simulink model "SpoolWrap"  (R2013b)
settings: Solver=ode3  StartTime=0.0  StopTime=5  FixedStep=.001  RelTol=1e-3
libraries: simulink x3
settings Model: Creator=LukePH  LastModifiedBy=LukePH

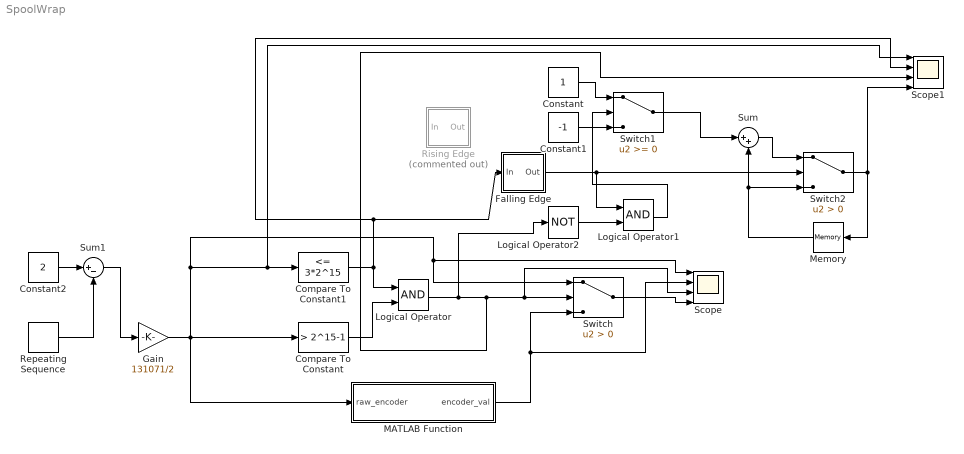
== system SpoolWrap ==
  Compare To Constant : simulink/Logic and Bit Operations/Compare To Constant  relop=>  const=2^15-1  OutDataTypeStr=boolean
  Compare To Constant1 : simulink/Logic and Bit Operations/Compare To Constant  relop=<=  const=3*2^15  OutDataTypeStr=boolean
  Constant : Constant
  Constant1 : Constant  Value=-1
  Constant2 : Constant  Value=2
  Falling Edge : Subsystem
  Gain : Gain  Gain=131071/2  OutDataTypeStr=int32
  Logical Operator : Logic  AllPortsSameDT=off  OutDataTypeStr=boolean
  Logical Operator1 : Logic  AllPortsSameDT=off  OutDataTypeStr=boolean
  Logical Operator2 : Logic  Operator=NOT  AllPortsSameDT=off  OutDataTypeStr=boolean
  MATLAB Function : MATLAB Function  TreatAsAtomicUnit=on
  Memory : Memory
  Repeating Sequence : simulink/Sources/Repeating Sequence  rep_seq_t=[0 1]  rep_seq_y=[0 2]
  Rising Edge : Subsystem  Commented=on
  Scope : Scope  NumInputPorts=4
      settings: TimeRange=4  YMin=0~-70000~0~-40000  YMax=140000~70000~1~100000
  Scope1 : Scope  NumInputPorts=4
      settings: TimeRange=4  YMin=0~-5~-5~-5  YMax=140000~5~5~5
  Sum : Sum  Inputs=|++
  Sum1 : Sum  Inputs=|+-
  Switch : Switch  Criteria=u2 > Threshold
  Switch1 : Switch
  Switch2 : Switch  Criteria=u2 > Threshold
  wires:
  Repeating Sequence/1 -> Sum1/2
  Gain/1 -> Scope/1, Switch/1, Scope1/1, Compare To Constant1/1, Compare To Constant/1, MATLAB Function/1(raw_encoder)
  Compare To Constant/1 -> Logical Operator/2
  Switch/1 -> Scope/4
  MATLAB Function/1(encoder_val) -> Scope/2, Switch/3
  Switch2/1 -> Memory/1, Scope1/4
  Memory/1 -> Sum/2, Switch2/3
  Constant1/1 -> Switch1/3
  Constant/1 -> Switch1/1
  Sum/1 -> Switch2/1
  Switch1/1 -> Sum/1
  Logical Operator/1 -> Logical Operator2/1, Scope1/3, Scope/3, Switch/2
  Falling Edge/1(Out) -> Logical Operator1/1, Switch2/2
  Compare To Constant1/1 -> Logical Operator/1, Falling Edge/1(In), Scope1/2
  Logical Operator1/1 -> Switch1/2
  Logical Operator2/1 -> Logical Operator1/2
  Constant2/1 -> Sum1/1
  Sum1/1 -> Gain/1

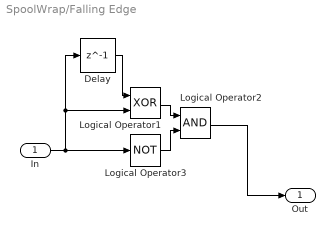
== system SpoolWrap/Falling Edge ==
  In : Inport
  Delay : Delay  DelayLength=1  InitialCondition=0
  Logical Operator1 : Logic  Operator=XOR  AllPortsSameDT=off  OutDataTypeStr=boolean
  Logical Operator2 : Logic  AllPortsSameDT=off  OutDataTypeStr=boolean
  Logical Operator3 : Logic  Operator=NOT  AllPortsSameDT=off  OutDataTypeStr=boolean
  Out : Outport
  wires:
  Delay/1 -> Logical Operator1/1
  Logical Operator1/1 -> Logical Operator2/1
  Logical Operator3/1 -> Logical Operator2/2
  Logical Operator2/1 -> Out/1
  In/1 -> Logical Operator3/1, Logical Operator1/2, Delay/1

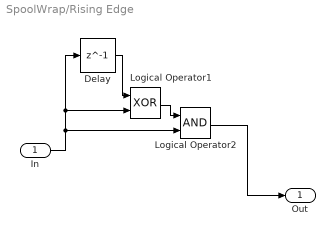
== system SpoolWrap/Rising Edge ==
  In : Inport
  Delay : Delay  DelayLength=1  InitialCondition=1
  Logical Operator1 : Logic  Operator=XOR  AllPortsSameDT=off  OutDataTypeStr=boolean
  Logical Operator2 : Logic  AllPortsSameDT=off  OutDataTypeStr=boolean
  Out : Outport
  wires:
  Logical Operator2/1 -> Out/1
  In/1 -> Logical Operator2/2, Delay/1, Logical Operator1/2
  Logical Operator1/1 -> Logical Operator2/1
  Delay/1 -> Logical Operator1/1

== matlab function SpoolWrap/MATLAB Function ==
  data: raw_encoder input; encoder_val output
function encoder_val = fcn(raw_encoder)
%#codegen

x = int32([0:65535,-65536:-1]);

encoder_val = x(int32(raw_encoder)+1);

end
